simulink model "test"  (R2026a)
settings: Solver=ode1  StopTime=300  FixedStep=10
settings Model: Creator=fofr6825  LastModifiedBy=fofr6825
settings DebuggingCC: InheritedTsInSrcMsg=none

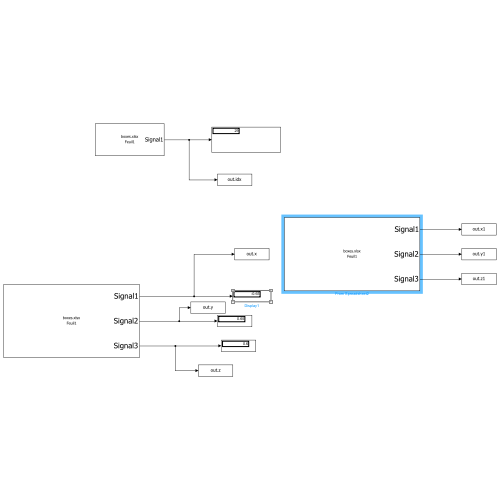
[thumbnail: Simulink's stored preview of the top-level diagram]
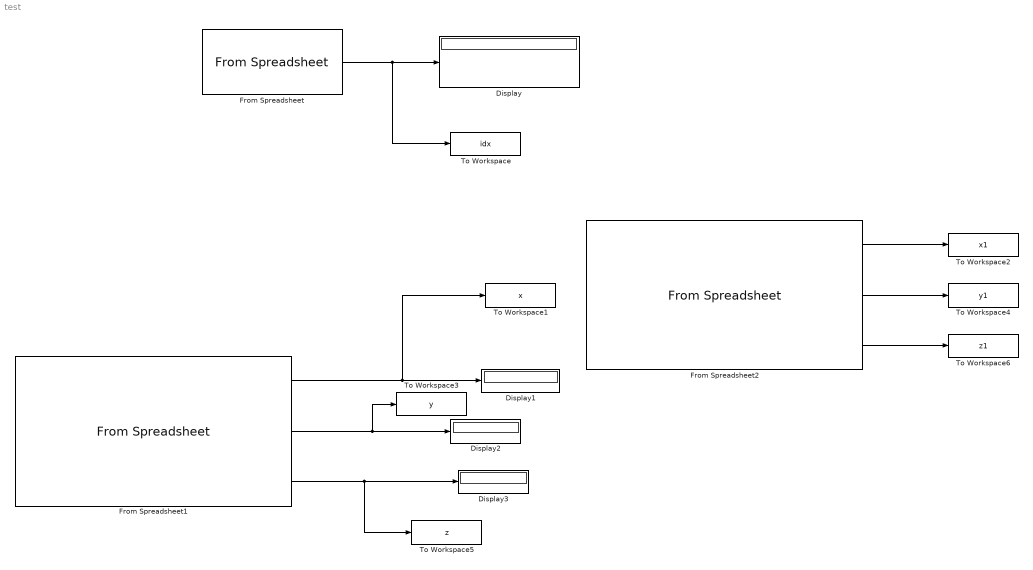
== system test ==
  Display{,1..3} (4 alike) : Display
  From Spreadsheet : FromSpreadsheet  FileName=boxes.xlsx  SheetName=Feuil1  Range=A2:A31  TreatFirstColumnAs=Data  SampleTime=-1  OutputAfterLastPoint=Hold final value
  From Spreadsheet1 : FromSpreadsheet  FileName=boxes.xlsx  SheetName=Feuil1  Range=A3:A31, F3:H31  SampleTime=-1
  From Spreadsheet2 : FromSpreadsheet  FileName=boxes.xlsx  SheetName=Feuil1  Range=A3:A31, B3:D31  SampleTime=-1
  To Workspace : ToWorkspace  VariableName=idx  SaveFormat=Timeseries  SampleTime=-1
  To Workspace1 : ToWorkspace  VariableName=x  SaveFormat=Timeseries  SampleTime=-1
  To Workspace2 : ToWorkspace  VariableName=x1  SaveFormat=Timeseries  SampleTime=-1
  To Workspace3 : ToWorkspace  VariableName=y  SaveFormat=Timeseries  SampleTime=-1
  To Workspace4 : ToWorkspace  VariableName=y1  SaveFormat=Timeseries  SampleTime=-1
  To Workspace5 : ToWorkspace  VariableName=z  SaveFormat=Timeseries  SampleTime=-1
  To Workspace6 : ToWorkspace  VariableName=z1  SaveFormat=Timeseries  SampleTime=-1
  wires:
  From Spreadsheet/1 -> To Workspace/1, Display/1
  From Spreadsheet1/2 -> To Workspace3/1, Display2/1
  From Spreadsheet1/3 -> To Workspace5/1, Display3/1
  From Spreadsheet1/1 -> To Workspace1/1, Display1/1
  From Spreadsheet2/1 -> To Workspace2/1
  From Spreadsheet2/2 -> To Workspace4/1
  From Spreadsheet2/3 -> To Workspace6/1
